simulink model "fail_driveline_mass"  (R2016b)
settings: Solver=ode4  StartTime=0.0  StopTime=10.0  FixedStep=0.01  RelTol=1e-3
libraries: fl_lib x6, nesl_utility x3
settings Model: TunableVars=A  TunableVarsStorageClass=Auto  Creator=jgillis  LastModifiedBy=jgillis
settings OptimizationCC: EnableMemcpy=off
settings RTWCC: RTWVerbose=off
settings SimscapeCC: SimscapeLogType=all  SimscapeLogLimitData=off  SimscapeLogDataHistory=1000

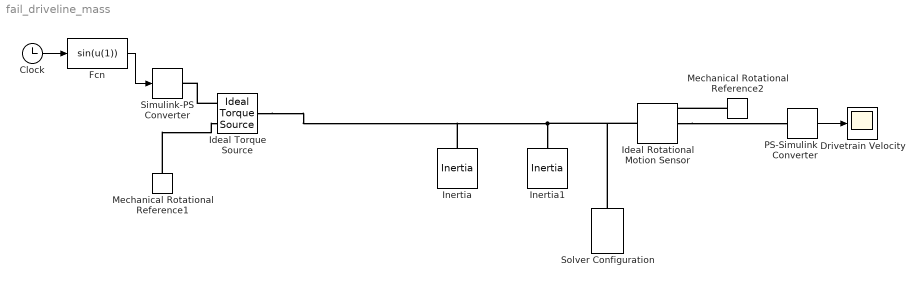
== system fail_driveline_mass ==
  Clock : Clock
  Drivetrain Velocity : Scope
  Fcn : Fcn  Expr=sin(u(1))
  Ideal Rotational Motion Sensor : fl_lib/Mechanical/Mechanical Sensors/Ideal Rotational Motion Sensor  offset=0 rad
  Ideal Torque Source : fl_lib/Mechanical/Mechanical Sources/Ideal Torque Source
  Inertia : fl_lib/Mechanical/Rotational Elements/Inertia  inertia=1 kg*m^2  w_specify=off  w_priority=High  w=0 rad/s  t_specify=off  t_priority=None  t=0 N*m
  Inertia1 : fl_lib/Mechanical/Rotational Elements/Inertia  inertia=9 kg*m^2  w_specify=off  w_priority=High  w=0 rad/s  t_specify=off  t_priority=None  t=0 N*m
  Mechanical Rotational Reference1 : fl_lib/Mechanical/Rotational Elements/Mechanical Rotational Reference
  Mechanical Rotational Reference2 : fl_lib/Mechanical/Rotational Elements/Mechanical Rotational Reference
  PS-Simulink Converter : nesl_utility/PS-Simulink Converter  PhysicalDomain=network_engine_domain  SubClassName=ps_output  LeftPortType=input  RightPortType=output  PseudoPeriodic=off  Frequencies=[]  Unit=1  AffineConversion=off
  Simulink-PS Converter : nesl_utility/Simulink-PS Converter  PhysicalDomain=network_engine_domain  SubClassName=ps_input  LeftPortType=input  RightPortType=output  PseudoPeriodic=off  Frequencies=[]  NoiseDistribution=none  NoiseParameters=[]  Unit=1  AffineConversion=off  InputFiltering=off  SimscapeFilterOrder=1  InputFilterTimeConstant=0.001  UdotUserProvided=1
  Solver Configuration : nesl_utility/Solver Configuration  PhysicalDomain=network_engine_domain  SubClassName=solver  LeftPortType=input  RightPortType=generic  Accelerate=off  Tones=[]  Harmonics=[]  SimulateNoise=off  Profile=off  UseLocalSampling=off  EnableSwitchedLinearOptims=on  FrequencyDomain=off  UseCCode=off  RelTol=0.001  AbsTol=1e-06  MinStep=1e-09  ToWorkspace=off  RevertToSquareIcSolve=off  NumHomotopyIterations=100  PhasorMode=off  PhasorModeNumHarmonics=1  OverrideAbsTol=off  DoDC=off  ResidualTolerance=1e-9  UseLocalSolver=on  LocalSolverChoice=NE_BACKWARD_EULER_ADVANCER  LocalSolverSampleTime=0.01  DoFixedCost=on  MaxNonlinIter=10  MaxModeIter=2  LinearAlgebra=Sparse  DelaysMemoryBudget=1024  AutomaticFiltering=on  FilteringTimeConstant=0.001
  wires:
  Clock/1 -> Fcn/1
  Fcn/1 -> Simulink-PS Converter/1
  PS-Simulink Converter/1 -> Drivetrain Velocity/1
  connections:
  Ideal Torque Source/RConn1 -- Simulink-PS Converter/RConn1
  Ideal Rotational Motion Sensor/LConn1 -- Solver Configuration/RConn1 -- Ideal Torque Source/LConn1 -- Inertia/LConn1 -- Inertia1/LConn1
  Ideal Rotational Motion Sensor/RConn2 -- PS-Simulink Converter/LConn1
  Mechanical Rotational Reference1/LConn1 -- Ideal Torque Source/RConn2
  Mechanical Rotational Reference2/LConn1 -- Ideal Rotational Motion Sensor/RConn1
